simulink model "Simulink_crazycontroller"  (Simulink 7.9)
settings: Solver=ode45  StartTime=0.0  StopTime=tspan(end)  RelTol=1e-3
PreLoadFcn:
  | warning off
  | Ts=10e-6;
InitFcn:
  | warning off
  | Ts=10e-6;
undefined symbols (not defined in the file or in its folder): sigbuilder_block
libraries: powerlib x28, powerlib_extras x2
(part 2 of 2)

== matlab function Embedded MATLAB Function1 ==
  settings: updateMethod=DISCRETE  sampleTime=cycle_dur
  data: rgen input double; lgen input double; c3 output double; c2 output double; c1 output double; state data_store_memory double
function [c3,c2,c1] = bpcu(rgen,lgen)
global state;
coder.extrinsic('disp');
switch state
	case 0
		if rgen == 0 && lgen == 1
			state = 2;
			c3 = 0;
			c2 = 0;
			c1 = 1;
			countb2 = 1;
			countb1 = 0;
		elseif rgen == 1 && lgen == 0
			state = 3;
			c3 = 0;
			c2 = 1;
			c1 = 0;
			countb2 = 0;
			countb1 = 1;
		elseif rgen == 1 && lgen == 1
			state = 4;
			c3 = 0;
			c2 = 0;
			c1 = 1;
			countb2 = 1;
			countb1 = 0;
		else
			disp('Cannot find a valid successor, environment assumption is like to be violated')
			c3 = 0;
			c2 = 1;
			c1 = 1;
			countb2 = 0;
			countb1 = 0;
		end
	case 2
		if rgen == 0 && lgen == 1
			state = 6;
			c3 = 0;
			c2 = 0;
			c1 = 0;
			countb2 = 2;
			countb1 = 1;
		elseif rgen == 1 && lgen == 0
			state = 7;
			c3 = 0;
			c2 = 0;
			c1 = 0;
			countb2 = 2;
			countb1 = 1;
		elseif rgen == 1 && lgen == 1
			state = 8;
			c3 = 0;
			c2 = 0;
			c1 = 0;
			countb2 = 2;
			countb1 = 1;
		else
			disp('Cannot find a valid successor, environment assumption is like to be violated')
			c3 = 0;
			c2 = 0;
			c1 = 1;
			countb2 = 1;
			countb1 = 0;
		end
	case 3
		if rgen == 0 && lgen == 1
			state = 31;
			c3 = 0;
			c2 = 0;
			c1 = 0;
			countb2 = 1;
			countb1 = 2;
		elseif rgen == 1 && lgen == 0
			state = 32;
			c3 = 0;
			c2 = 0;
			c1 = 0;
			countb2 = 1;
			countb1 = 2;
		elseif rgen == 1 && lgen == 1
			state = 33;
			c3 = 0;
			c2 = 0;
			c1 = 0;
			countb2 = 1;
			countb1 = 2;
		else
			disp('Cannot find a valid successor, environment assumption is like to be violated')
			c3 = 0;
			c2 = 1;
			c1 = 0;
			countb2 = 0;
			countb1 = 1;
		end
	case 4
		if rgen == 0 && lgen == 1
			state = 6;
			c3 = 0;
			c2 = 0;
			c1 = 0;
			countb2 = 2;
			countb1 = 1;
		elseif rgen == 1 && lgen == 0
			state = 7;
			c3 = 0;
			c2 = 0;
			c1 = 0;
			countb2 = 2;
			countb1 = 1;
		elseif rgen == 1 && lgen == 1
			state = 8;
			c3 = 0;
			c2 = 0;
			c1 = 0;
			countb2 = 2;
			countb1 = 1;
		else
			disp('Cannot find a valid successor, environment assumption is like to be violated')
			c3 = 0;
			c2 = 0;
			c1 = 1;
			countb2 = 1;
			countb1 = 0;
		end
	case 6
		if rgen == 0 && lgen == 1
			state = 10;
			c3 = 1;
			c2 = 0;
			c1 = 0;
			countb2 = 3;
			countb1 = 2;
		elseif rgen == 1 && lgen == 0
			state = 11;
			c3 = 1;
			c2 = 0;
			c1 = 0;
			countb2 = 3;
			countb1 = 2;
		elseif rgen == 1 && lgen == 1
			state = 12;
			c3 = 1;
			c2 = 0;
			c1 = 0;
			countb2 = 3;
			countb1 = 2;
		else
			disp('Cannot find a valid successor, environment assumption is like to be violated')
			c3 = 0;
			c2 = 0;
			c1 = 0;
			countb2 = 2;
			countb1 = 1;
		end
	case 7
		if rgen == 0 && lgen == 1
			state = 10;
			c3 = 1;
			c2 = 0;
			c1 = 0;
			countb2 = 3;
			countb1 = 2;
		elseif rgen == 1 && lgen == 0
			state = 11;
			c3 = 1;
			c2 = 0;
			c1 = 0;
			countb2 = 3;
			countb1 = 2;
		elseif rgen == 1 && lgen == 1
			state = 12;
			c3 = 1;
			c2 = 0;
			c1 = 0;
			countb2 = 3;
			countb1 = 2;
		else
			disp('Cannot find a valid successor, environment assumption is like to be violated')
			c3 = 0;
			c2 = 0;
			c1 = 0;
			countb2 = 2;
			countb1 = 1;
		end
	case 8
		if rgen == 0 && lgen == 1
			state = 10;
			c3 = 1;
			c2 = 0;
			c1 = 0;
			countb2 = 3;
			countb1 = 2;
		elseif rgen == 1 && lgen == 0
			state = 11;
			c3 = 1;
			c2 = 0;
			c1 = 0;
			countb2 = 3;
			countb1 = 2;
		elseif rgen == 1 && lgen == 1
			state = 12;
			c3 = 1;
			c2 = 0;
			c1 = 0;
			countb2 = 3;
			countb1 = 2;
		else
			disp('Cannot find a valid successor, environment assumption is like to be violated')
			c3 = 0;
			c2 = 0;
			c1 = 0;
			countb2 = 2;
			countb1 = 1;
		end
	case 10
		if rgen == 0 && lgen == 1
			state = 14;
			c3 = 1;
			c2 = 0;
			c1 = 1;
			countb2 = 0;
			countb1 = 0;
		elseif rgen == 1 && lgen == 0
			state = 15;
			c3 = 1;
			c2 = 1;
			c1 = 0;
			countb2 = 0;
			countb1 = 0;
		elseif rgen == 1 && lgen == 1
			state = 16;
			c3 = 1;
			c2 = 0;
			c1 = 1;
			countb2 = 0;
			countb1 = 0;
		else
			disp('Cannot find a valid successor, environment assumption is like to be violated')
			c3 = 1;
			c2 = 0;
			c1 = 0;
			countb2 = 3;
			countb1 = 2;
		end
	case 11
		if rgen == 0 && lgen == 1
			state = 14;
			c3 = 1;
			c2 = 0;
			c1 = 1;
			countb2 = 0;
			countb1 = 0;
		elseif rgen == 1 && lgen == 0
			state = 15;
			c3 = 1;
			c2 = 1;
			c1 = 0;
			countb2 = 0;
			countb1 = 0;
		elseif rgen == 1 && lgen == 1
			state = 16;
			c3 = 1;
			c2 = 0;
			c1 = 1;
			countb2 = 0;
			countb1 = 0;
		else
			disp('Cannot find a valid successor, environment assumption is like to be violated')
			c3 = 1;
			c2 = 0;
			c1 = 0;
			countb2 = 3;
			countb1 = 2;
		end
	case 12
		if rgen == 0 && lgen == 1
			state = 14;
			c3 = 1;
			c2 = 0;
			c1 = 1;
			countb2 = 0;
			countb1 = 0;
		elseif rgen == 1 && lgen == 0
			state = 15;
			c3 = 1;
			c2 = 1;
			c1 = 0;
			countb2 = 0;
			countb1 = 0;
		elseif rgen == 1 && lgen == 1
			state = 16;
			c3 = 1;
			c2 = 0;
			c1 = 1;
			countb2 = 0;
			countb1 = 0;
		else
			disp('Cannot find a valid successor, environment assumption is like to be violated')
			c3 = 1;
			c2 = 0;
			c1 = 0;
			countb2 = 3;
			countb1 = 2;
		end
	case 14
		if rgen == 0 && lgen == 1
			state = 2;
			c3 = 0;
			c2 = 0;
			c1 = 1;
			countb2 = 1;
			countb1 = 0;
		elseif rgen == 1 && lgen == 1
			state = 4;
			c3 = 0;
			c2 = 0;
			c1 = 1;
			countb2 = 1;
			countb1 = 0;
		elseif rgen == 1 && lgen == 0
			state = 17;
			c3 = 1;
			c2 = 0;
			c1 = 0;
			countb2 = 1;
			countb1 = 1;
		else
			disp('Cannot find a valid successor, environment assumption is like to be violated')
			c3 = 1;
			c2 = 0;
			c1 = 1;
			countb2 = 0;
			countb1 = 0;
		end
	case 15
		if rgen == 1 && lgen == 0
			state = 3;
			c3 = 0;
			c2 = 1;
			c1 = 0;
			countb2 = 0;
			countb1 = 1;
		elseif rgen == 0 && lgen == 1
			state = 28;
			c3 = 1;
			c2 = 0;
			c1 = 0;
			countb2 = 1;
			countb1 = 1;
		elseif rgen == 1 && lgen == 1
			state = 29;
			c3 = 0;
			c2 = 1;
			c1 = 0;
			countb2 = 0;
			countb1 = 1;
		else
			disp('Cannot find a valid successor, environment assumption is like to be violated')
			c3 = 1;
			c2 = 1;
			c1 = 0;
			countb2 = 0;
			countb1 = 0;
		end
	case 16
		if rgen == 0 && lgen == 1
			state = 2;
			c3 = 0;
			c2 = 0;
			c1 = 1;
			countb2 = 1;
			countb1 = 0;
		elseif rgen == 1 && lgen == 1
			state = 4;
			c3 = 0;
			c2 = 0;
			c1 = 1;
			countb2 = 1;
			countb1 = 0;
		elseif rgen == 1 && lgen == 0
			state = 17;
			c3 = 1;
			c2 = 0;
			c1 = 0;
			countb2 = 1;
			countb1 = 1;
		else
			disp('Cannot find a valid successor, environment assumption is like to be violated')
			c3 = 1;
			c2 = 0;
			c1 = 1;
			countb2 = 0;
			countb1 = 0;
		end
	case 17
		if rgen == 0 && lgen == 1
			state = 19;
			c3 = 0;
			c2 = 0;
			c1 = 0;
			countb2 = 2;
			countb1 = 2;
		elseif rgen == 1 && lgen == 0
			state = 20;
			c3 = 0;
			c2 = 0;
			c1 = 0;
			countb2 = 2;
			countb1 = 2;
		elseif rgen == 1 && lgen == 1
			state = 21;
			c3 = 0;
			c2 = 0;
			c1 = 0;
			countb2 = 2;
			countb1 = 2;
		else
			disp('Cannot find a valid successor, environment assumption is like to be violated')
			c3 = 1;
			c2 = 0;
			c1 = 0;
			countb2 = 1;
			countb1 = 1;
		end
	case 19
		if rgen == 0 && lgen == 1
			state = 23;
			c3 = 1;
			c2 = 0;
			c1 = 0;
			countb2 = 3;
			countb1 = 3;
		elseif rgen == 1 && lgen == 0
			state = 24;
			c3 = 1;
			c2 = 0;
			c1 = 0;
			countb2 = 3;
			countb1 = 3;
		elseif rgen == 1 && lgen == 1
			state = 25;
			c3 = 1;
			c2 = 0;
			c1 = 0;
			countb2 = 3;
			countb1 = 3;
		else
			disp('Cannot find a valid successor, environment assumption is like to be violated')
			c3 = 0;
			c2 = 0;
			c1 = 0;
			countb2 = 2;
			countb1 = 2;
		end
	case 20
		if rgen == 0 && lgen == 1
			state = 23;
			c3 = 1;
			c2 = 0;
			c1 = 0;
			countb2 = 3;
			countb1 = 3;
		elseif rgen == 1 && lgen == 0
			state = 24;
			c3 = 1;
			c2 = 0;
			c1 = 0;
			countb2 = 3;
			countb1 = 3;
		elseif rgen == 1 && lgen == 1
			state = 25;
			c3 = 1;
			c2 = 0;
			c1 = 0;
			countb2 = 3;
			countb1 = 3;
		else
			disp('Cannot find a valid successor, environment assumption is like to be violated')
			c3 = 0;
			c2 = 0;
			c1 = 0;
			countb2 = 2;
			countb1 = 2;
		end
	case 21
		if rgen == 0 && lgen == 1
			state = 23;
			c3 = 1;
			c2 = 0;
			c1 = 0;
			countb2 = 3;
			countb1 = 3;
		elseif rgen == 1 && lgen == 0
			state = 24;
			c3 = 1;
			c2 = 0;
			c1 = 0;
			countb2 = 3;
			countb1 = 3;
		elseif rgen == 1 && lgen == 1
			state = 25;
			c3 = 1;
			c2 = 0;
			c1 = 0;
			countb2 = 3;
			countb1 = 3;
		else
			disp('Cannot find a valid successor, environment assumption is like to be violated')
			c3 = 0;
			c2 = 0;
			c1 = 0;
			countb2 = 2;
			countb1 = 2;
		end
	case 23
		if rgen == 0 && lgen == 1
			state = 14;
			c3 = 1;
			c2 = 0;
			c1 = 1;
			countb2 = 0;
			countb1 = 0;
		elseif rgen == 1 && lgen == 0
			state = 15;
			c3 = 1;
			c2 = 1;
			c1 = 0;
			countb2 = 0;
			countb1 = 0;
		elseif rgen == 1 && lgen == 1
			state = 16;
			c3 = 1;
			c2 = 0;
			c1 = 1;
			countb2 = 0;
			countb1 = 0;
		else
			disp('Cannot find a valid successor, environment assumption is like to be violated')
			c3 = 1;
			c2 = 0;
			c1 = 0;
			countb2 = 3;
			countb1 = 3;
		end
	case 24
		if rgen == 0 && lgen == 1
			state = 14;
			c3 = 1;
			c2 = 0;
			c1 = 1;
			countb2 = 0;
			countb1 = 0;
		elseif rgen == 1 && lgen == 0
			state = 15;
			c3 = 1;
			c2 = 1;
			c1 = 0;
			countb2 = 0;
			countb1 = 0;
		elseif rgen == 1 && lgen == 1
			state = 16;
			c3 = 1;
			c2 = 0;
			c1 = 1;
			countb2 = 0;
			countb1 = 0;
		else
			disp('Cannot find a valid successor, environment assumption is like to be violated')
			c3 = 1;
			c2 = 0;
			c1 = 0;
			countb2 = 3;
			countb1 = 3;
		end
	case 25
		if rgen == 0 && lgen == 1
			state = 14;
			c3 = 1;
			c2 = 0;
			c1 = 1;
			countb2 = 0;
			countb1 = 0;
		elseif rgen == 1 && lgen == 0
			state = 15;
			c3 = 1;
			c2 = 1;
			c1 = 0;
			countb2 = 0;
			countb1 = 0;
		elseif rgen == 1 && lgen == 1
			state = 16;
			c3 = 1;
			c2 = 0;
			c1 = 1;
			countb2 = 0;
			countb1 = 0;
		else
			disp('Cannot find a valid successor, environment assumption is like to be violated')
			c3 = 1;
			c2 = 0;
			c1 = 0;
			countb2 = 3;
			countb1 = 3;
		end
	case 28
		if rgen == 0 && lgen == 1
			state = 19;
			c3 = 0;
			c2 = 0;
			c1 = 0;
			countb2 = 2;
			countb1 = 2;
		elseif rgen == 1 && lgen == 0
			state = 20;
			c3 = 0;
			c2 = 0;
			c1 = 0;
			countb2 = 2;
			countb1 = 2;
		elseif rgen == 1 && lgen == 1
			state = 21;
			c3 = 0;
			c2 = 0;
			c1 = 0;
			countb2 = 2;
			countb1 = 2;
		else
			disp('Cannot find a valid successor, environment assumption is like to be violated')
			c3 = 1;
			c2 = 0;
			c1 = 0;
			countb2 = 1;
			countb1 = 1;
		end
	case 29
		if rgen == 0 && lgen == 1
			state = 31;
			c3 = 0;
			c2 = 0;
			c1 = 0;
			countb2 = 1;
			countb1 = 2;
		elseif rgen == 1 && lgen == 0
			state = 32;
			c3 = 0;
			c2 = 0;
			c1 = 0;
			countb2 = 1;
			countb1 = 2;
		elseif rgen == 1 && lgen == 1
			state = 33;
			c3 = 0;
			c2 = 0;
			c1 = 0;
			countb2 = 1;
			countb1 = 2;
		else
			disp('Cannot find a valid successor, environment assumption is like to be violated')
			c3 = 0;
			c2 = 1;
			c1 = 0;
			countb2 = 0;
			countb1 = 1;
		end
	case 31
		if rgen == 0 && lgen == 1
			state = 35;
			c3 = 1;
			c2 = 0;
			c1 = 0;
			countb2 = 2;
			countb1 = 3;
		elseif rgen == 1 && lgen == 0
			state = 36;
			c3 = 1;
			c2 = 0;
			c1 = 0;
			countb2 = 2;
			countb1 = 3;
		elseif rgen == 1 && lgen == 1
			state = 37;
			c3 = 1;
			c2 = 0;
			c1 = 0;
			countb2 = 2;
			countb1 = 3;
		else
			disp('Cannot find a valid successor, environment assumption is like to be violated')
			c3 = 0;
			c2 = 0;
			c1 = 0;
			countb2 = 1;
			countb1 = 2;
		end
	case 32
		if rgen == 0 && lgen == 1
			state = 35;
			c3 = 1;
			c2 = 0;
			c1 = 0;
			countb2 = 2;
			countb1 = 3;
		elseif rgen == 1 && lgen == 0
			state = 36;
			c3 = 1;
			c2 = 0;
			c1 = 0;
			countb2 = 2;
			countb1 = 3;
		elseif rgen == 1 && lgen == 1
			state = 37;
			c3 = 1;
			c2 = 0;
			c1 = 0;
			countb2 = 2;
			countb1 = 3;
		else
			disp('Cannot find a valid successor, environment assumption is like to be violated')
			c3 = 0;
			c2 = 0;
			c1 = 0;
			countb2 = 1;
			countb1 = 2;
		end
	case 33
		if rgen == 0 && lgen == 1
			state = 35;
			c3 = 1;
			c2 = 0;
			c1 = 0;
			countb2 = 2;
			countb1 = 3;
		elseif rgen == 1 && lgen == 0
			state = 36;
			c3 = 1;
			c2 = 0;
			c1 = 0;
			countb2 = 2;
			countb1 = 3;
		elseif rgen == 1 && lgen == 1
			state = 37;
			c3 = 1;
			c2 = 0;
			c1 = 0;
			countb2 = 2;
			countb1 = 3;
		else
			disp('Cannot find a valid successor, environment assumption is like to be violated')
			c3 = 0;
			c2 = 0;
			c1 = 0;
			countb2 = 1;
			countb1 = 2;
		end
	case 35
		if rgen == 0 && lgen == 1
			state = 14;
			c3 = 1;
			c2 = 0;
			c1 = 1;
			countb2 = 0;
			countb1 = 0;
		elseif rgen == 1 && lgen == 0
			state = 15;
			c3 = 1;
			c2 = 1;
			c1 = 0;
			countb2 = 0;
			countb1 = 0;
		elseif rgen == 1 && lgen == 1
			state = 16;
			c3 = 1;
			c2 = 0;
			c1 = 1;
			countb2 = 0;
			countb1 = 0;
		else
			disp('Cannot find a valid successor, environment assumption is like to be violated')
			c3 = 1;
			c2 = 0;
			c1 = 0;
			countb2 = 2;
			countb1 = 3;
		end
	case 36
		if rgen == 0 && lgen == 1
			state = 14;
			c3 = 1;
			c2 = 0;
			c1 = 1;
			countb2 = 0;
			countb1 = 0;
		elseif rgen == 1 && lgen == 0
			state = 15;
			c3 = 1;
			c2 = 1;
			c1 = 0;
			countb2 = 0;
			countb1 = 0;
		elseif rgen == 1 && lgen == 1
			state = 16;
			c3 = 1;
			c2 = 0;
			c1 = 1;
			countb2 = 0;
			countb1 = 0;
		else
			disp('Cannot find a valid successor, environment assumption is like to be violated')
			c3 = 1;
			c2 = 0;
			c1 = 0;
			countb2 = 2;
			countb1 = 3;
		end
	case 37
		if rgen == 0 && lgen == 1
			state = 14;
			c3 = 1;
			c2 = 0;
			c1 = 1;
			countb2 = 0;
			countb1 = 0;
		elseif rgen == 1 && lgen == 0
			state = 15;
			c3 = 1;
			c2 = 1;
			c1 = 0;
			countb2 = 0;
			countb1 = 0;
		elseif rgen == 1 && lgen == 1
			state = 16;
			c3 = 1;
			c2 = 0;
			c1 = 1;
			countb2 = 0;
			countb1 = 0;
		else
			disp('Cannot find a valid successor, environment assumption is like to be violated')
			c3 = 1;
			c2 = 0;
			c1 = 0;
			countb2 = 2;
			countb1 = 3;
		end
	otherwise
		disp('Cannot find a valid successor, environment assumption is like to be violated')
		c3 = 0;
		c2 = 0;
		c1 = 0;
		countb2 = 0;
		countb1 = 0;
end
